simulink model "Mmc"  (R2024b)
settings: Solver=ode23t  StartTime=0.0  StopTime=0.04  MaxStep=1e-6  RelTol=1e-3
values from neighbouring files (symbols this model uses):
  C_PM = 1e9    (= 1000000000)    [MmcParameters.m]
  Nb_PM = 20    [MmcParameters.m]
  Ts_Power = 10e-6    (= 1e-05)    [MmcParameters.m]
  VDCm = (Nb_PM * Vnom_PM) / 2    (= 10000)    [MmcParameters.m]
  VDCp = (Nb_PM * Vnom_PM) / 2    (= 10000)    [MmcParameters.m]
libraries: spsSeriesRLCBranchLib x8, spsHalfBridgeMMCLib x6, spsVoltageMeasurementLib x3, spsGroundLib x2, spsDCVoltageSourceLib x2, sps_lib x1
settings Model: Creator=The MathWorks, Inc.  LastModifiedBy=sct23
settings SolverCC: AlgebraicLoopSolver=TrustRegion
settings DataIOCC: SaveFormat=StructureWithTime  SaveOutput=off  SignalLogging=off  DSMLogging=off  SaveTime=off  ReturnWorkspaceOutputs=off
settings OptimizationCC: ExpressionDepthLimit=2147483647  LifeSpan=inf
settings DebuggingCC: UnderspecifiedInitializationDetection=Classic  MergeDetectMultiDrivingBlocksExec=none  SolverPrmCheckMsg=warning  FcnCallInpInsideContextMsg=warning  UnconnectedInputMsg=warning  UnconnectedOutputMsg=warning  UnconnectedLineMsg=warning  AllowSymbolicDim=off  StateNameClashWarn=warning  SFUnexpectedBacktrackingDiag=warning  SFNoUnconditionalDefaultTransitionDiag=warning  SFExecutionAtInitializationDiag=none  ArithmeticOperatorsInVariantConditions=warning
settings HardwareCC: ProdBitPerPointer=32  ProdBitPerSizeT=32  ProdBitPerPtrDiffT=32  ProdLargestAtomicFloat=None  ProdIntDivRoundTo=Undefined  ProdEndianess=Unspecified  ProdWordSize=32  ProdHWDeviceType=32-bit Generic
settings ModelReferenceCC: EnableRefExpFcnMdlSchedulingChecks=on  PropagateSignalLabelsOutOfModel=off
settings SFSimCC: SimUseLocalCustomCode=off  CustomCodeUndefinedFunction=UseInterfaceOnly
settings RTWCC: RTWUseLocalCustomCode=off  GPUComputeCapability=3.5
settings CodeAppCC: StateflowObjectComments=on
settings GRTTargetCC: TargetLangStandard=C89/C90 (ANSI)  CombineOutputUpdateFcns=off  GRTInterface=on
settings ConfigComp: CovMetricSettings=dw  CovSaveCumulativeToWorkspaceVar=on  CovSaveSingleToWorkspaceVar=on  CovExternalEMLEnable=off
settings SimscapeCC: SimscapeNormalizeSystem=off  SimscapeNominalValues={1, 'bar'; 1, 'cm^3/s'; 1, 'bar*kg/s'; 1, 'kJ/kg'; 1, 'kW'; }

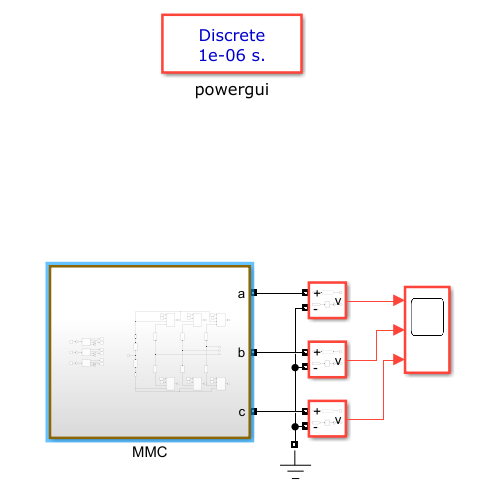
[thumbnail: Simulink's stored preview of the top-level diagram]
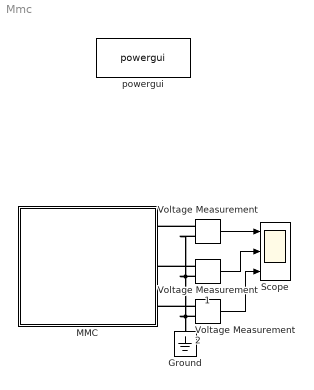
== system Mmc ==
  Ground : spsGroundLib/Ground  LConnTagsString=a
  MMC : Subsystem
  Scope : Scope  NumInputPorts=3
  Voltage Measurement : spsVoltageMeasurementLib/Voltage Measurement  PhasorSimulation=off  OutputType=Complex  PSBequivalent=0
  Voltage Measurement1 : spsVoltageMeasurementLib/Voltage Measurement  PhasorSimulation=off  OutputType=Complex  PSBequivalent=0
  Voltage Measurement2 : spsVoltageMeasurementLib/Voltage Measurement  PhasorSimulation=off  OutputType=Complex  PSBequivalent=0
  powergui : sps_lib/powergui  Priority=1  SimulationMode=Discrete  SampleTime=1e-6  frequency=60  Iterations=50  frequencyindice=0  Pbase=100e6  ErrMax=1e-4  UnitsV=kV  UnitsW=MW  buscounter=0  FunctionMessages=off  echomessages=off  EnableUseOfTLC=off  CurrentSourceSwitches=off  DisableSnubberDevices=off  DisableRonSwitches=off  DisableVfSwitches=off  DisplayEquations=off  AutomaticDiscreteSolvers=off  SolverType=Tustin/Backward Euler (TBE)  Interpol=off  ExternalGateDelay=off  methode=off  Ts=10  x0status=blocks  SPID=off  SwTol=0  HookPort=off  NonlinearTolerance=1e-4  nMaxIteration=100  ContinueOnMaxIteration=off  RestoreLinks=warning  ResistiveCurrentMeasurement=off  Frange=[0:2:500]  Ylog=off  Xlog=on  ShowGrid=off  save=off  variable=ZData  structure=Vout  ZoomFFT=on  StartTime=0.15  cycles=2  DisplayStyle=1  fundamental=50  FreqAxis=on  MaxFrequency=6000  frequencyindicesteady=1  RmsSteady=1  display=off
  wires:
  Voltage Measurement/1 -> Scope/1
  Voltage Measurement1/1 -> Scope/2
  Voltage Measurement2/1 -> Scope/3
  connections:
  Voltage Measurement/LConn1 -- MMC/LConn1
  Voltage Measurement/LConn2 -- Voltage Measurement1/LConn2 -- Voltage Measurement2/LConn2 -- Ground/LConn1
  Voltage Measurement1/LConn1 -- MMC/LConn2
  Voltage Measurement2/LConn1 -- MMC/LConn3

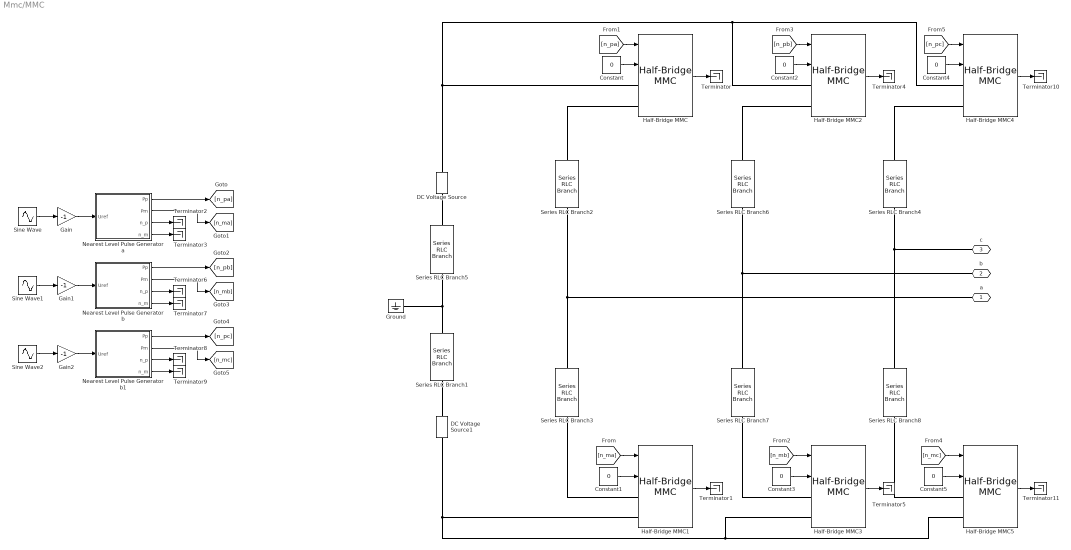
== system Mmc/MMC ==
  Constant{,1..5} (6 alike) : Constant  Value=0
  DC Voltage Source : spsDCVoltageSourceLib/DC Voltage Source  Amplitude=VDCp  Measurements=None
  DC Voltage Source1 : spsDCVoltageSourceLib/DC Voltage Source  Amplitude=VDCm  Measurements=None
  Gain : Gain  Gain=-1
  Gain1 : Gain  Gain=-1
  Gain2 : Gain  Gain=-1
  Ground : spsGroundLib/Ground  LConnTagsString=a
  Half-Bridge MMC{,1..5} (6 alike) : spsHalfBridgeMMCLib/Half-Bridge MMC  ModelType=Switching devices  n=Nb_PM  C=C_PM  Vc_Initial=Vc_Initial  Ron=Ron  Rs=Rs  Cs=Cs  Ron_Diode=1e-3  Rs_Diode=1e6  Cs_Diode=inf  Vf_Diode=1e-3  Rs_CurrentSource=inf  Ts=10e-6
      settings: LibrarySourceBlock=sps_lib/Power Electronics/Half-Bridge MMC
  "Nearest Level Pulse Generator a " : Subsystem
  Nearest Level Pulse Generator b : Subsystem
  Nearest Level Pulse Generator b1 : Subsystem
  Series RLC Branch{1..8} (8 alike) : spsSeriesRLCBranchLib/Series RLC Branch  LConnTagsString=__new0  RConnTagsString=__new0  BranchType=RL  Resistance=.1  Inductance=1e-3  SetiL0=off  InitialCurrent=0  Capacitance=1e-6  Setx0=off  InitialVoltage=0  Measurements=None
  Sine Wave : Sin  Frequency=2*pi*50  SampleTime=Ts_Power
  Sine Wave1 : Sin  Frequency=2*pi*50  Phase=4*pi/3  SampleTime=Ts_Power
  Sine Wave2 : Sin  Frequency=2*pi*50  Phase=2*pi/3  SampleTime=Ts_Power
  Terminator{,1..11} (12 alike) : Terminator
  a : PMIOPort  Side=Left
  b : PMIOPort  Port=2  Side=Left
  c : PMIOPort  Port=3  Side=Left
  wires:
  Constant4/1 -> Half-Bridge MMC4/2
  Gain1/1 -> Nearest Level Pulse Generator b/1(Uref)
  [n_pc] -> Half-Bridge MMC4/1
  [n_pb] -> Half-Bridge MMC2/1
  [n_pa] -> Half-Bridge MMC/1
  Sine Wave/1 -> Gain/1
  Nearest Level Pulse Generator b/1(Pp) -> [n_pb]
  Nearest Level Pulse Generator b/2(Pm) -> [n_mb]
  Nearest Level Pulse Generator b1/4(n_m) -> Terminator9/1
  [n_mb] -> Half-Bridge MMC3/1
  Constant1/1 -> Half-Bridge MMC1/2
  Sine Wave2/1 -> Gain2/1
  Nearest Level Pulse Generator b1/3(n_p) -> Terminator8/1
  "Nearest Level Pulse Generator a "/2(Pm) -> [n_ma]
  Gain/1 -> "Nearest Level Pulse Generator a "/1(Uref)
  Nearest Level Pulse Generator b1/2(Pm) -> [n_mc]
  Gain2/1 -> Nearest Level Pulse Generator b1/1(Uref)
  Sine Wave1/1 -> Gain1/1
  Half-Bridge MMC3/1 -> Terminator5/1
  Constant3/1 -> Half-Bridge MMC3/2
  Nearest Level Pulse Generator b1/1(Pp) -> [n_pc]
  "Nearest Level Pulse Generator a "/4(n_m) -> Terminator3/1
  Half-Bridge MMC/1 -> Terminator/1
  Nearest Level Pulse Generator b/4(n_m) -> Terminator7/1
  Nearest Level Pulse Generator b/3(n_p) -> Terminator6/1
  Half-Bridge MMC5/1 -> Terminator11/1
  Half-Bridge MMC2/1 -> Terminator4/1
  "Nearest Level Pulse Generator a "/1(Pp) -> [n_pa]
  Constant2/1 -> Half-Bridge MMC2/2
  Constant/1 -> Half-Bridge MMC/2
  [n_ma] -> Half-Bridge MMC1/1
  Constant5/1 -> Half-Bridge MMC5/2
  "Nearest Level Pulse Generator a "/3(n_p) -> Terminator2/1
  Half-Bridge MMC1/1 -> Terminator1/1
  Half-Bridge MMC4/1 -> Terminator10/1
  [n_mc] -> Half-Bridge MMC5/1
  connections:
  Series RLC Branch1/RConn1 -- DC Voltage Source1/RConn1
  DC Voltage Source1/LConn1 -- Half-Bridge MMC5/LConn2 -- Half-Bridge MMC3/LConn2 -- Half-Bridge MMC1/LConn2
  Series RLC Branch4/LConn1 -- Half-Bridge MMC4/LConn2
  DC Voltage Source/RConn1 -- Half-Bridge MMC/LConn1 -- Half-Bridge MMC2/LConn1 -- Half-Bridge MMC4/LConn1
  Series RLC Branch8/LConn1 -- c/RConn1 -- Series RLC Branch4/RConn1
  Series RLC Branch1/LConn1 -- Series RLC Branch5/RConn1 -- Ground/LConn1
  Series RLC Branch2/LConn1 -- Half-Bridge MMC/LConn2
  Series RLC Branch7/RConn1 -- Half-Bridge MMC3/LConn1
  Series RLC Branch3/LConn1 -- a/RConn1 -- Series RLC Branch2/RConn1
  Series RLC Branch6/LConn1 -- Half-Bridge MMC2/LConn2
  Series RLC Branch8/RConn1 -- Half-Bridge MMC5/LConn1
  Series RLC Branch3/RConn1 -- Half-Bridge MMC1/LConn1
  Series RLC Branch7/LConn1 -- b/RConn1 -- Series RLC Branch6/RConn1
  Series RLC Branch5/LConn1 -- DC Voltage Source/LConn1

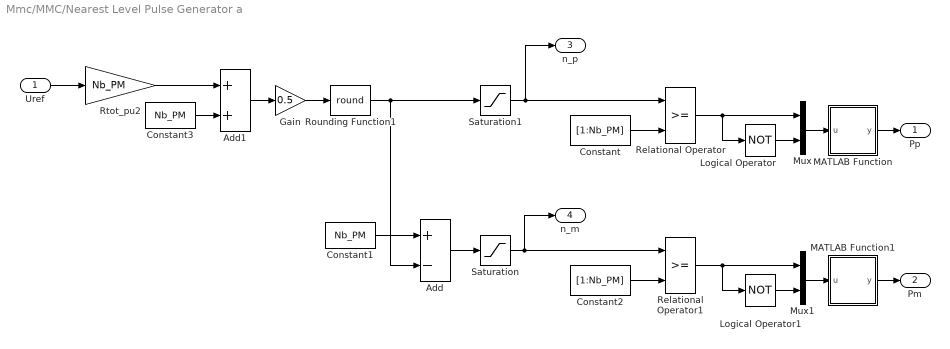
== system Mmc/MMC/Nearest Level Pulse Generator a  ==
  Uref : Inport
  Add : Sum  Inputs=+-
  Add1 : Sum
  Constant : Constant  Value=[1:Nb_PM]
  Constant1 : Constant  Value=Nb_PM
  Constant2 : Constant  Value=[1:Nb_PM]
  Constant3 : Constant  Value=Nb_PM
  Gain : Gain  Gain=0.5
  Logical Operator : Logic  Operator=NOT  AllPortsSameDT=off  OutDataTypeStr=float('double')
  Logical Operator1 : Logic  Operator=NOT  AllPortsSameDT=off  OutDataTypeStr=float('double')
  MATLAB Function : MATLAB Function  TreatAsAtomicUnit=on
  MATLAB Function1 : MATLAB Function  TreatAsAtomicUnit=on
  Mux : Mux  Inputs=2
  Mux1 : Mux  Inputs=2
  Relational Operator : RelationalOperator  OutDataTypeStr=float('double')  InputSameDT=off
  Relational Operator1 : RelationalOperator  OutDataTypeStr=float('double')  InputSameDT=off
  Rounding Function1 : Rounding  Operator=round
  Rtot_pu2 : Gain  Gain=Nb_PM  SaturateOnIntegerOverflow=on  OutDataTypeStr=Inherit: Same as input  ParamDataTypeStr=Inherit: Same as input
  Saturation : Saturate  UpperLimit=Nb_PM  LowerLimit=0
  Saturation1 : Saturate  UpperLimit=Nb_PM  LowerLimit=0
  Pp : Outport  VectorParamsAs1DForOutWhenUnconnected=off
  Pm : Outport  Port=2  VectorParamsAs1DForOutWhenUnconnected=off
  n_p : Outport  Port=3  VectorParamsAs1DForOutWhenUnconnected=off
  n_m : Outport  Port=4  VectorParamsAs1DForOutWhenUnconnected=off
  wires:
  Constant/1 -> Relational Operator/2
  Relational Operator/1 -> Logical Operator/1, Mux/1
  Logical Operator/1 -> Mux/2
  Mux/1 -> MATLAB Function/1(u)
  MATLAB Function/1(y) -> Pp/1
  Add/1 -> Saturation/1
  Constant1/1 -> Add/1
  Saturation1/1 -> n_p/1, Relational Operator/1
  Rtot_pu2/1 -> Add1/1
  Constant3/1 -> Add1/2
  Add1/1 -> Gain/1
  Gain/1 -> Rounding Function1/1
  Rounding Function1/1 -> Add/2, Saturation1/1
  Uref/1 -> Rtot_pu2/1
  Constant2/1 -> Relational Operator1/2
  Relational Operator1/1 -> Mux1/1, Logical Operator1/1
  Logical Operator1/1 -> Mux1/2
  Mux1/1 -> MATLAB Function1/1(u)
  MATLAB Function1/1(y) -> Pm/1
  Saturation/1 -> n_m/1, Relational Operator1/1

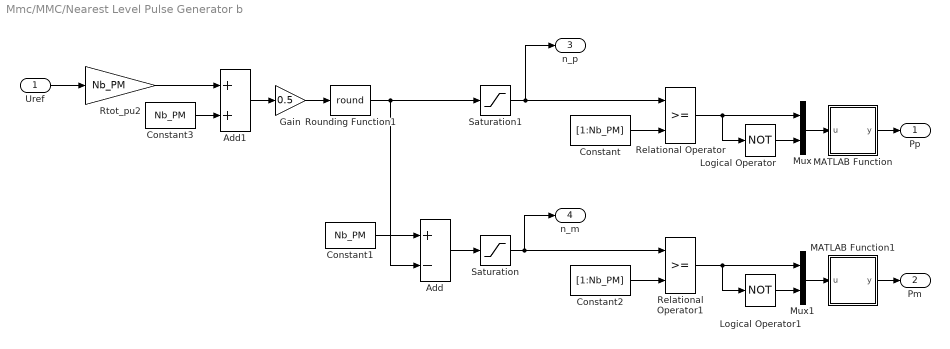
== system Mmc/MMC/Nearest Level Pulse Generator b ==
  Uref : Inport
  Add : Sum  Inputs=+-
  Add1 : Sum
  Constant : Constant  Value=[1:Nb_PM]
  Constant1 : Constant  Value=Nb_PM
  Constant2 : Constant  Value=[1:Nb_PM]
  Constant3 : Constant  Value=Nb_PM
  Gain : Gain  Gain=0.5
  Logical Operator : Logic  Operator=NOT  AllPortsSameDT=off  OutDataTypeStr=float('double')
  Logical Operator1 : Logic  Operator=NOT  AllPortsSameDT=off  OutDataTypeStr=float('double')
  MATLAB Function : MATLAB Function  TreatAsAtomicUnit=on
  MATLAB Function1 : MATLAB Function  TreatAsAtomicUnit=on
  Mux : Mux  Inputs=2
  Mux1 : Mux  Inputs=2
  Relational Operator : RelationalOperator  OutDataTypeStr=float('double')  InputSameDT=off
  Relational Operator1 : RelationalOperator  OutDataTypeStr=float('double')  InputSameDT=off
  Rounding Function1 : Rounding  Operator=round
  Rtot_pu2 : Gain  Gain=Nb_PM  SaturateOnIntegerOverflow=on  OutDataTypeStr=Inherit: Same as input  ParamDataTypeStr=Inherit: Same as input
  Saturation : Saturate  UpperLimit=Nb_PM  LowerLimit=0
  Saturation1 : Saturate  UpperLimit=Nb_PM  LowerLimit=0
  Pp : Outport  VectorParamsAs1DForOutWhenUnconnected=off
  Pm : Outport  Port=2  VectorParamsAs1DForOutWhenUnconnected=off
  n_p : Outport  Port=3  VectorParamsAs1DForOutWhenUnconnected=off
  n_m : Outport  Port=4  VectorParamsAs1DForOutWhenUnconnected=off
  wires:
  Constant/1 -> Relational Operator/2
  Relational Operator/1 -> Logical Operator/1, Mux/1
  Logical Operator/1 -> Mux/2
  Mux/1 -> MATLAB Function/1(u)
  MATLAB Function/1(y) -> Pp/1
  Add/1 -> Saturation/1
  Constant1/1 -> Add/1
  Saturation1/1 -> n_p/1, Relational Operator/1
  Rtot_pu2/1 -> Add1/1
  Constant3/1 -> Add1/2
  Add1/1 -> Gain/1
  Gain/1 -> Rounding Function1/1
  Rounding Function1/1 -> Add/2, Saturation1/1
  Uref/1 -> Rtot_pu2/1
  Constant2/1 -> Relational Operator1/2
  Relational Operator1/1 -> Mux1/1, Logical Operator1/1
  Logical Operator1/1 -> Mux1/2
  Mux1/1 -> MATLAB Function1/1(u)
  MATLAB Function1/1(y) -> Pm/1
  Saturation/1 -> n_m/1, Relational Operator1/1

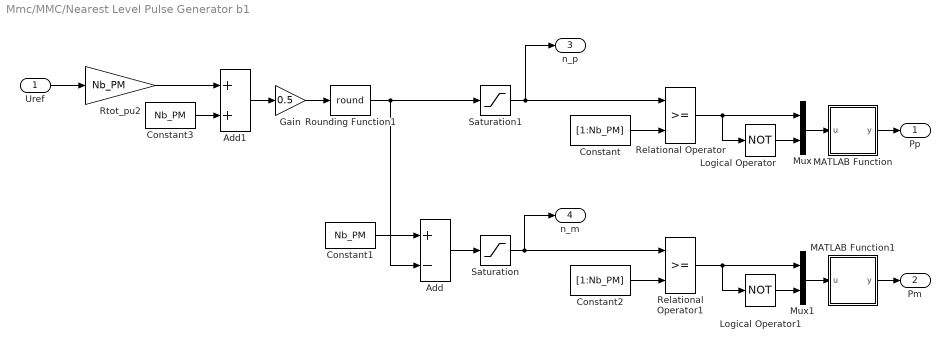
== system Mmc/MMC/Nearest Level Pulse Generator b1 ==
  Uref : Inport
  Add : Sum  Inputs=+-
  Add1 : Sum
  Constant : Constant  Value=[1:Nb_PM]
  Constant1 : Constant  Value=Nb_PM
  Constant2 : Constant  Value=[1:Nb_PM]
  Constant3 : Constant  Value=Nb_PM
  Gain : Gain  Gain=0.5
  Logical Operator : Logic  Operator=NOT  AllPortsSameDT=off  OutDataTypeStr=float('double')
  Logical Operator1 : Logic  Operator=NOT  AllPortsSameDT=off  OutDataTypeStr=float('double')
  MATLAB Function : MATLAB Function  TreatAsAtomicUnit=on
  MATLAB Function1 : MATLAB Function  TreatAsAtomicUnit=on
  Mux : Mux  Inputs=2
  Mux1 : Mux  Inputs=2
  Relational Operator : RelationalOperator  OutDataTypeStr=float('double')  InputSameDT=off
  Relational Operator1 : RelationalOperator  OutDataTypeStr=float('double')  InputSameDT=off
  Rounding Function1 : Rounding  Operator=round
  Rtot_pu2 : Gain  Gain=Nb_PM  SaturateOnIntegerOverflow=on  OutDataTypeStr=Inherit: Same as input  ParamDataTypeStr=Inherit: Same as input
  Saturation : Saturate  UpperLimit=Nb_PM  LowerLimit=0
  Saturation1 : Saturate  UpperLimit=Nb_PM  LowerLimit=0
  Pp : Outport  VectorParamsAs1DForOutWhenUnconnected=off
  Pm : Outport  Port=2  VectorParamsAs1DForOutWhenUnconnected=off
  n_p : Outport  Port=3  VectorParamsAs1DForOutWhenUnconnected=off
  n_m : Outport  Port=4  VectorParamsAs1DForOutWhenUnconnected=off
  wires:
  Constant/1 -> Relational Operator/2
  Relational Operator/1 -> Logical Operator/1, Mux/1
  Logical Operator/1 -> Mux/2
  Mux/1 -> MATLAB Function/1(u)
  MATLAB Function/1(y) -> Pp/1
  Add/1 -> Saturation/1
  Constant1/1 -> Add/1
  Saturation1/1 -> n_p/1, Relational Operator/1
  Rtot_pu2/1 -> Add1/1
  Constant3/1 -> Add1/2
  Add1/1 -> Gain/1
  Gain/1 -> Rounding Function1/1
  Rounding Function1/1 -> Add/2, Saturation1/1
  Uref/1 -> Rtot_pu2/1
  Constant2/1 -> Relational Operator1/2
  Relational Operator1/1 -> Mux1/1, Logical Operator1/1
  Logical Operator1/1 -> Mux1/2
  Mux1/1 -> MATLAB Function1/1(u)
  MATLAB Function1/1(y) -> Pm/1
  Saturation/1 -> n_m/1, Relational Operator1/1

== matlab function Mmc/MMC/Nearest Level Pulse Generator a /MATLAB Function ==
  data: u input; y output
function y = FiringSorting(u)
    y = u;
    for i = 1: length(u)
        if mod(i, 2) == 1
            y(i) = u(int16(i/2));
        else
            y(i) = u(int16(i/2+length(u)/2));
        end
    end
end

== matlab function Mmc/MMC/Nearest Level Pulse Generator b/MATLAB Function ==
  data: u input; y output
function y = FiringSorting(u)
    y = u;
    for i = 1: length(u)
        if mod(i, 2) == 1
            y(i) = u(int16(i/2));
        else
            y(i) = u(int16(i/2+length(u)/2));
        end
    end
end

== matlab function Mmc/MMC/Nearest Level Pulse Generator b/MATLAB Function1 ==
  data: u input; y output
function y = FiringSorting(u)
    y = u;
    for i = 1: length(u)
        if mod(i, 2) == 1
            y(i) = u(int16(i/2));
        else
            y(i) = u(int16(i/2+length(u)/2));
        end
    end
end

== matlab function Mmc/MMC/Nearest Level Pulse Generator b1/MATLAB Function ==
  data: u input; y output
function y = FiringSorting(u)
    y = u;
    for i = 1: length(u)
        if mod(i, 2) == 1
            y(i) = u(int16(i/2));
        else
            y(i) = u(int16(i/2+length(u)/2));
        end
    end
end

== matlab function Mmc/MMC/Nearest Level Pulse Generator b1/MATLAB Function1 ==
  data: u input; y output
function y = FiringSorting(u)
    y = u;
    for i = 1: length(u)
        if mod(i, 2) == 1
            y(i) = u(int16(i/2));
        else
            y(i) = u(int16(i/2+length(u)/2));
        end
    end
end

== matlab function Mmc/MMC/Nearest Level Pulse Generator a /MATLAB Function1 ==
  data: u input; y output
function y = FiringSorting(u)
    y = u;
    for i = 1: length(u)
        if mod(i, 2) == 1
            y(i) = u(int16(i/2));
        else
            y(i) = u(int16(i/2+length(u)/2));
        end
    end
end
